simulink model "PubIfDecisionLSM_MDL"  (R2020b)
settings: configuration reference "DspaceConfig" (kept outside this file)
PostLoadFcn:
  | if any(exist('dsrtsu_mdlpostloadfcn', 'file') ~= 0), dsrtsu_mdlpostloadfcn('Execute', bdroot); end
InitFcn:
  | , if any(exist('rtifpga_mdlclblib', 'file') ~= 0), rtifpga_mdlclblib('Init', bdroot); end,
  | , if any(exist('dsmpb_private', 'file') ~= 0), dsmpb_private('dsmpb_mdlclblib', 'Init', bdroot); end,
values from neighbouring files (symbols this model uses):
  P_LSM_ALC_Enable = 0.0    [LSM_Parameter.sldd]
  P_LSM_AwayEdge_offset = 0.1    [LSM_Parameter.sldd]
  P_LSM_CentValidErr = 1.0    [LSM_Parameter.sldd]
  P_LSM_DOP_C0_EN_Limit = 0.8    [LSM_Parameter.sldd]
  P_LSM_DOP_C0_out_Limit = 2.0    [LSM_Parameter.sldd]
  P_LSM_DOP_C1_EN_Limit : value not decoded    [LSM_Parameter.sldd]
  P_LSM_DOP_C1_out_Limit : value not decoded    [LSM_Parameter.sldd]
  P_LSM_DOP_C1AndC2_Lim_X : value not decoded    [LSM_Parameter.sldd]
  P_LSM_DOP_C2_EN_Limit : value not decoded    [LSM_Parameter.sldd]
  P_LSM_DOP_C2_out_Limit : value not decoded    [LSM_Parameter.sldd]
  P_LSM_DOP_In_Pre2Dop_Dis = 1.0    [LSM_Parameter.sldd]
  P_LSM_DOP_Out_Pre2Dop_Dis = 2.0    [LSM_Parameter.sldd]
  P_LSM_DOP_PreDis_X : value not decoded    [LSM_Parameter.sldd]
  P_LSM_DOP_PreDis_Y : value not decoded    [LSM_Parameter.sldd]
  P_LSM_DOPEnableSW = 1.0    [LSM_Parameter.sldd]
  P_LSM_DOPValid_CheckTime = 0.06    [LSM_Parameter.sldd]
  P_LSM_DoubleLine_Curr2Cent_Dislimit = 0.5    [LSM_Parameter.sldd]
  P_LSM_DoubleLine_Dop2Cent_Dislimit = 0.5    [LSM_Parameter.sldd]
  P_LSM_DoubleLine_DOPOut_C1 : value not decoded    [LSM_Parameter.sldd]
  P_LSM_DoubleLine_Pre2Cent_Dislimit = 1.0    [LSM_Parameter.sldd]
  P_LSM_Error_Limit = 0.5    [LSM_Parameter.sldd]
  P_LSM_IFV2CenterAxis = 0.0    [LSM_Parameter.sldd]
  P_LSM_IFV2RearAxis = 0.0    [LSM_Parameter.sldd]
  P_LSM_Line2Edge_limit = 0.5    [LSM_Parameter.sldd]
  P_LSM_Line_Error = 0.1    [LSM_Parameter.sldd]
  P_LSM_LineSTD_Limit = 0.15    [LSM_Parameter.sldd]
  P_LSM_NOH_Switch = 0.0    [LSM_Parameter.sldd]
  P_LSM_OTL_C0_Factor = 1.0    [LSM_Parameter.sldd]
  P_LSM_OTL_C1_Factor = 0.5    [LSM_Parameter.sldd]
  P_LSM_OTL_C2_Factor = 0.5    [LSM_Parameter.sldd]
  P_LSM_Pre2OnlyLineDis = 5.0    [LSM_Parameter.sldd]
  P_LSM_Pre_t = 0.0    [LSM_Parameter.sldd]
  P_LSM_SingleLine_Cent2Edge_Dislimit = 100.0    [LSM_Parameter.sldd]
  P_LSM_SingleLine_Curr2Cent_Dislimit = 0.2    [LSM_Parameter.sldd]
  P_LSM_SingleLine_Dop2Cent_Dislimit = 0.2    [LSM_Parameter.sldd]
  P_LSM_SingleLine_DOPOut_C1 : value not decoded    [LSM_Parameter.sldd]
  P_LSM_SingleLine_Pre2Cent_Dislimit = 0.5    [LSM_Parameter.sldd]
  P_LSM_TJALimitSpd = 60.0    [LSM_Parameter.sldd]
undefined symbols (not defined in the file or in its folder): P_lCS_IFV2CenterAxis, P_LCS_IFV2RearAxis, P_LSM_EntryEdge_offset, P_LSM_EntryLnChngEnSwitch, P_LSM_EntryVanishDis, P_LSM_LinetLostTime, P_LSM_LineWijCal_C12, P_LSM_LineWijCal_C13, P_LSM_MapValid_ErrorSwitch, P_LSM_PosLineLcFac, P_LSM_SpdLim_Stub_Spd, P_LSM_SpdLim_StubLength, P_LSM_SpdTurnAlarm
libraries: simulink x324, TrueDurationTime x11
(part 10 of 25)

== system PubIfDecisionLSM_MDL/Subsystem1/TargetLineCalc_20ms2/TargetLineCalc/Subsystem3 ==
  Intersec_available : Inport  OutDataTypeStr=uint8
  f_distance : Inport  Port=2  OutDataTypeStr=single
  f_end_dis : Inport  Port=3
  en_direction : Inport  Port=4  OutDataTypeStr=uint8
  i_rec_lanes_num : Inport  Port=5  OutDataTypeStr=uint8
  i_rec_lanes : Inport  Port=6  OutDataTypeStr=uint8
  nLaneNum : Inport  Port=7  OutDataTypeStr=uint8
  nLaneID : Inport  Port=8  OutDataTypeStr=uint8
  i_mapvalid : Inport  Port=9  OutDataTypeStr=uint8
  i_on_nav_path : Inport  Port=10  OutDataTypeStr=uint8
  curr_b_vanish_valid : Inport  Port=11  OutDataTypeStr=boolean
  Exit_dDisStart : Inport  Port=12  OutDataTypeStr=single
  ExitLineExist : Inport  Port=13  OutDataTypeStr=uint8
  Exit_dC0V : Inport  Port=14  OutDataTypeStr=single
  RoadType : Inport  Port=15  OutDataTypeStr=uint8
  VehInLeftmostLane : Inport  Port=16  OutDataTypeStr=boolean
  VehInRightmostLane : Inport  Port=17  OutDataTypeStr=boolean
  Entry_bIsLineExist : Inport  Port=18
  Entry_dDisStart : Inport  Port=19
  Entry_dC0V : Inport  Port=20
  "curr_f_vanish_pt_dis " : Inport  Port=21
  currentLane_type : Inport  Port=22
  currentLane_valid : Inport  Port=23
  ChgSpd_Dis : Inport  Port=24
  SpdChgMax : Inport  Port=25
  rightLane_valid : Inport  Port=26
  rightLane_type : Inport  Port=27
  right_b_vanish_valid : Inport  Port=28
  right_f_vanish_pt_dis : Inport  Port=29
  leftLane_valid : Inport  Port=30
  leftLane_type : Inport  Port=31
  left_b_vanish_valid : Inport  Port=32
  " left_f_vanish_pt_dis" : Inport  Port=33
  RFM_ODD : Inport  Port=34  OutDataTypeStr=Bus: RFM_ODD_BUS  PortDimensions=1  BusOutputAsStruct=on
  NOH_Sts : Inport  Port=35
  vehSpd : Inport  Port=36
  Double_Line_Lost : Inport  Port=37
  HWASts : Inport  Port=38
  KapTraj : Inport  Port=39
  VxvRef : Inport  Port=40
  TarLineValid : Inport  Port=41
  TarLineA3 : Inport  Port=42
  TarLineA2 : Inport  Port=43
  TarLineA1 : Inport  Port=44
  TarLineA0 : Inport  Port=45
  Chart1 : Stateflow chart  TreatAsAtomicUnit=on
  EgoLineRef : Subsystem
  HWASts1 : InportShadow  Port=38
  Signal Copy{,1..8,13,16..17} (12 alike) : SignalConversion  OverrideOpt=off
  Subsystem : Subsystem
  Subsystem1 : Subsystem
  Subsystem2 : Subsystem
  Subsystem3 : Subsystem
  Subsystem4 : Subsystem
  Terminator : Terminator
  Unit Delay : UnitDelay  SampleTime=-1  HasFrameUpgradeWarning=on
  VehInRightmostLane1 : InportShadow  Port=17  OutDataTypeStr=boolean
  nLaneNum1 : InportShadow  Port=7  OutDataTypeStr=uint8
  nLaneNum2 : InportShadow  Port=7  OutDataTypeStr=uint8
  PilotRoadSts : Outport  OutDataTypeStr=uint8
  PilotTurnSwSts : Outport  Port=2  OutDataTypeStr=uint8
  PilotSts : Outport  Port=3  OutDataTypeStr=uint8
  LaneChange : Outport  Port=4  OutDataTypeStr=uint8
  LSM_PilotSPL : Outport  Port=5  OutDataTypeStr=uint8
  PilotSPLDist : Outport  Port=6  OutDataTypeStr=uint16
  LSM_PilotNohExitDist : Outport  Port=7
  NOH_HMI_Voice : Outport  Port=8
  wires:
  SpdChgMax/1 -> Subsystem/45(SpdChgMax)
  ChgSpd_Dis/1 -> Subsystem/44(ChgSpd_Dis)
  Signal Copy8/1 -> Subsystem2/7(VehInRightmostLane)
  Signal Copy7/1 -> Chart1/6(vehSpd)  "LSM_VehSpd_HiFlag"
  Signal Copy6/1 -> Subsystem4/11(LaneNum)
  Chart1/3(m) -> Terminator/1  "LSM_TurnHighSpdFlag"
  HWASts1/1 -> Subsystem2/31(HWASts)
  EgoLineRef/1(LaneChangeEnable) -> Subsystem/48(LaneChangeEnable)
  TarLineA0/1 -> EgoLineRef/7(TarLineA0)
  TarLineA1/1 -> EgoLineRef/6(TarLineA1)
  TarLineA2/1 -> EgoLineRef/5(TarLineA2)
  TarLineA3/1 -> EgoLineRef/4(TarLineA3)
  TarLineValid/1 -> EgoLineRef/3(TarLineValid)
  VxvRef/1 -> EgoLineRef/2(VxvRef)
  KapTraj/1 -> EgoLineRef/1(KapTraj)
  Subsystem2/36(EntryStubVanishTurn) -> Subsystem/41(EntryStubVanishTurn)
  [f_distance] -> Subsystem/4(f_distance)
  [f_distance] -> Subsystem1/5(f_distance)
  Subsystem4/1(NOH_HMI_Voice) -> NOH_HMI_Voice/1
  HWASts/1 -> Subsystem4/14(HWASts)
  [NoPUCR_Dis] -> Subsystem4/13(NoPUCR_Dis)
  [NoPUCR] -> Subsystem4/12(NoPUCR)
  nLaneNum1/1 -> Signal Copy6/1
  Double_Line_Lost/1 -> Subsystem4/10(Double_Line_Lost)
  [f_distance] -> Subsystem4/9(f_distance)
  [rExitStub4_takeover] -> Subsystem4/8(rExitStub4_takeover)
  [lExitStub4_takeover] -> Subsystem4/7(lExitStub4_takeover)
  [exitTakeOverValid] -> Subsystem4/6(exitTakeOverValid)
  [b_vanish_valid] -> Subsystem4/5(b_vanish_valid)
  [changeVoice] -> Subsystem4/4(changeVoice)
  [f_vanish_pt_dis] -> Subsystem4/3(f_vanish_pt_dis)
  [en_direction] -> Subsystem4/2(en_direction)
  [PilotRoadSts] -> Subsystem4/1(PilotRoadSts)
  [NoPUCR] -> Subsystem1/4(NoPUCR)
  Subsystem2/35(StudLengthSpd) -> Subsystem/40(StudLengthSpd)
  [vehSpd] -> Subsystem/47(vehSpd)
  Subsystem2/34(ForbidActive) -> Subsystem/39(ForbidActive)
  currentLane_valid/1 -> Subsystem2/30(currentLane_valid)
  Subsystem2/33(DecSpd) -> Subsystem/38(DecSpd)
  Subsystem/8(NoPUCR_Dis) -> [NoPUCR_Dis]
  Subsystem/7(NoPUCR) -> [NoPUCR]
  Subsystem2/37(exitTakeOverValid) -> [exitTakeOverValid]
  [vehSpd] -> Signal Copy7/1
  Signal Copy13/1 -> Subsystem/42(RFM_ODD)
  Signal Copy17/1 -> Subsystem2/23(VehSpd), [vehSpd]
  Signal Copy16/1 -> Chart1/5(nLaneNum)  "LSM_nLaneNum_HiFlag"
  Signal Copy5/1 -> Chart1/4(VehInRightmostLane)  "LSM_MostLaneRight_HiFlag"
  Subsystem/1(PilotRoadSts) -> PilotRoadSts/1, Chart1/1(PilotRoadSts), Unit Delay/1, [PilotRoadSts]
  Chart1/2(changeVoice) -> [changeVoice]
  vehSpd/1 -> Signal Copy17/1
  nLaneNum2/1 -> Signal Copy16/1
  VehInRightmostLane1/1 -> Signal Copy5/1
  Unit Delay/1 -> Chart1/2(PilotRoadSts_K)
  Chart1/1(PilotTurnSwSts) -> PilotTurnSwSts/1, [PilotTurnSwSts]
  Subsystem2/32(roadClass) -> Subsystem/37(roadClass)
  currentLane_type/1 -> Subsystem2/22(currentLane_type)
  leftLane_type/1 -> Subsystem2/21(leftLane_type)
  rightLane_type/1 -> Subsystem2/19(rightLane_type)
  Subsystem/6(LSM_PilotNohExitDist) -> LSM_PilotNohExitDist/1
  RFM_ODD/1 -> Signal Copy13/1
  leftLane_valid/1 -> Subsystem2/20(leftLane_valid)
  rightLane_valid/1 -> Subsystem2/18(rightLane_valid)
  Subsystem2/31(turndir) -> Subsystem/36(turndir)
  Signal Copy2/1 -> Subsystem2/1(Exit_bIsLineExist), Subsystem/5(bIsLineExist)
  Signal Copy4/1 -> [f_distance], Subsystem2/2(f_distance)
  Signal Copy3/1 -> Subsystem1/3(RoadType)
  Signal Copy1/1 -> Subsystem1/2(i_on_nav_path)
  Signal Copy/1 -> Subsystem1/1(i_mapvalid)
  f_distance/1 -> Signal Copy4/1
  RoadType/1 -> Signal Copy3/1
  [nLaneID] -> Subsystem3/2(nLaneID)
  [PilotTurnSwSts] -> Subsystem3/1(PilotTurnSwSts)
  Subsystem/5(PilotSts) -> PilotSts/1
  Subsystem2/30(Vanish_turnleft_takeover) -> Subsystem/35(Vanish_turnleft_takeover)
  Subsystem2/29(EntryStub5_takeover) -> Subsystem/34(EntryStub5_takeover)  "LSM_EntryStub5_takeover"
  Subsystem2/28(lExitStub4_takeover) -> [lExitStub4_takeover], Subsystem/33(lExitStub4_takeover)
  Subsystem2/27(rExitStub4_takeover) -> Subsystem/32(rExitStub4_takeover), [rExitStub4_takeover]
  Subsystem3/1(LaneChange) -> LaneChange/1
  "curr_f_vanish_pt_dis "/1 -> Subsystem2/17(" curr_f_vanish_pt_dis "), [f_vanish_pt_dis]
  Subsystem/4(PilotSPLDist) -> PilotSPLDist/1
  Subsystem/3(LSM_PilotSPL) -> LSM_PilotSPL/1
  Subsystem2/26(EntryStub5_TurnLeft) -> Subsystem/31(EntryStub5_TurnLeft)
  Subsystem2/25(EntryStub6) -> Subsystem/30(EntryStub6)  "LSM_EntryStub6"
  Subsystem2/24(EntryStub5) -> Subsystem/29(EntryStub5)  "LSM_EntryStub5"
  Subsystem2/23(EntryStub4) -> Subsystem/28(EntryStub4)  "LSM_EntryStub4"
  Subsystem2/22(EntryStub3) -> Subsystem/27(EntryStub3)  "LSM_EntryStub3"
  Subsystem2/21(EntryStub2) -> Subsystem/26(EntryStub2)  "LSM_EntryStub2"
  Subsystem2/20(OneLane) -> Subsystem/25(OneLane)  "LSM_OneLane"
  Subsystem2/19(Forbid_TurnLeft) -> Subsystem/24(FrbLeft)
  Subsystem2/18(Forbid_TurnRight) -> Subsystem/23(FrbRight)
  Subsystem2/17(CruiseTurn) -> Subsystem/22(CruiseTurn)  "LSM_CruiseTurn"
  Subsystem2/15(lExitStub2) -> Subsystem/20(lExitStub2)  "LSM_IExitStub2"
  Subsystem2/14(lExitStub1) -> Subsystem/19(lExitStub1)  "LSM_IExitStub1"
  Subsystem2/13(CruiseLeft) -> Subsystem/18(CruiseLeft)  "LSM_CruiseLeft"
  Subsystem2/12(CruiseRight) -> Subsystem/17(CruiseRight)  "LSM_CruiseRight"
  Subsystem2/11(EntryStub1) -> Subsystem/16(EntryStub1)  "LSM_EntryStub1"
  Subsystem2/10(Vanish_turnleft) -> Subsystem/15(Vanish_turnleft)  "LSM_Vanish_turnleft"
  Subsystem2/8(rExitStub2) -> Subsystem/13(rExitStub2)  "LSM_rExitStub2"
  Subsystem2/7(rExitStub1) -> Subsystem/12(rExitStub1)  "LSM_rExitStub1"
  Subsystem2/6(TurnRight) -> Subsystem/11(TurnRight)  "LSM_TurnRight"
  Subsystem2/5(TurnLeft) -> Subsystem/10(TurnLeft)  "LSM_TurnLeft"
  Subsystem2/4(CruiseValid) -> Subsystem/9(CruiseValid)  "LSM_CruiseValid"
  Subsystem2/3(LeftStub) -> Subsystem/8(LeftStub)  "LSM_LeftStub"
  Subsystem2/2(RightStub) -> Subsystem/7(RightStub)  "LSM_RightStub"
  Subsystem2/1(StubValid) -> Subsystem/6(StubValid)  "LSM_StubValid"
  Subsystem/2(PilotTurnSwSts) -> Chart1/3(PilotTurnSwSts_Init)
  Entry_dC0V/1 -> [Entry_dC0V], Subsystem2/16(Entry_dC0V)
  Entry_dDisStart/1 -> Subsystem2/15(Entry_dDisStart)
  Entry_bIsLineExist/1 -> Subsystem2/14(Entry_bIsLineExist)
  Intersec_available/1 -> Subsystem2/3(b_is_available)
  Subsystem2/16(lExitStub3) -> Subsystem/21(lExitStub3)  "LSM_IExitStub3"
  en_direction/1 -> Subsystem2/6(en_direction), [en_direction]
  ExitLineExist/1 -> Signal Copy2/1
  i_rec_lanes/1 -> Subsystem2/4(i_rec_lanes)
  i_mapvalid/1 -> Signal Copy/1
  i_rec_lanes_num/1 -> Subsystem2/10(i_rec_lanes_num)
  Subsystem2/9(rExitStub3) -> Subsystem/14(rExitStub3)  "LSM_rExitStub3"
  Exit_dDisStart/1 -> Subsystem2/12(" Exit_dDisStart")
  Exit_dC0V/1 -> Subsystem2/13(Exit_dC0V)
  i_on_nav_path/1 -> Signal Copy1/1
  nLaneID/1 -> Subsystem2/5(nLaneID), [nLaneID]
  VehInRightmostLane/1 -> Signal Copy8/1
  VehInLeftmostLane/1 -> Subsystem2/8(VehInLeftmostLane)
  nLaneNum/1 -> Subsystem2/9(nLaneNum)
  curr_b_vanish_valid/1 -> Subsystem2/11(" curr_b_vanish_valid"), [b_vanish_valid]
  f_end_dis/1 -> Subsystem2/24(f_end_dis)
  [PilotRoadSts] -> Subsystem2/25(PilotRoadSts)
  left_b_vanish_valid/1 -> Subsystem2/26(left_b_vanish_valid)
  " left_f_vanish_pt_dis"/1 -> Subsystem2/27(" left_f_vanish_pt_dis")
  right_b_vanish_valid/1 -> Subsystem2/28(right_b_vanish_valid)
  right_f_vanish_pt_dis/1 -> Subsystem2/29(right_f_vanish_pt_dis)
  Subsystem1/1(i_mapvalid_out) -> Subsystem/1(i_mapvalid)
  Subsystem1/2(i_on_nav_path_out) -> Subsystem/2(i_on_nav_path)
  Subsystem1/3(RoadType_out) -> Subsystem/3(RoadType)
  NOH_Sts/1 -> Subsystem/43(NOH_Sts)
  [Entry_dC0V] -> Subsystem/46(Entry_dC0V)

== system PubIfDecisionLSM_MDL/Subsystem1/TargetLineCalc_20ms2/TargetLineCalc/TypeConf ==
  LeftType : Inport
  LeftDLMType : Inport  Port=2
  LeftDECELType : Inport  Port=3
  RightType : Inport  Port=4
  RightDLMType : Inport  Port=5
  RightDECELType : Inport  Port=6
  RoadWidthCalc1 : MATLAB Function  TreatAsAtomicUnit=on
  Unit Delay36 : UnitDelay  SampleTime=-1  HasFrameUpgradeWarning=on
  Unit Delay37 : UnitDelay  SampleTime=-1  HasFrameUpgradeWarning=on
  Out1 : Outport
  Out2 : Outport  Port=2
  wires:
  RightDECELType/1 -> RoadWidthCalc1/6(RightDECELType)
  LeftDECELType/1 -> RoadWidthCalc1/3(LeftDECELType)
  RightDLMType/1 -> RoadWidthCalc1/5(RightDLMType)
  LeftDLMType/1 -> RoadWidthCalc1/2(LeftDLMType)
  RightType/1 -> RoadWidthCalc1/4(RightType)
  Unit Delay36/1 -> RoadWidthCalc1/8(Cnt2K1)
  RoadWidthCalc1/2(RightEn) -> Out2/1
  LeftType/1 -> RoadWidthCalc1/1(LeftType)
  RoadWidthCalc1/4(Cnt2) -> Unit Delay36/1
  RoadWidthCalc1/3(Cnt1) -> Unit Delay37/1
  Unit Delay37/1 -> RoadWidthCalc1/7(Cnt1K1)
  RoadWidthCalc1/1(LeftEn) -> Out1/1

== system PubIfDecisionLSM_MDL/Subsystem1/TargetLineCalc_20ms2/TargetLineCalc/TypeConf1 ==
  LeftType : Inport
  RightType : Inport  Port=2
  RoadWidthCalc1 : MATLAB Function  TreatAsAtomicUnit=on
  Unit Delay36 : UnitDelay  SampleTime=-1  HasFrameUpgradeWarning=on
  Unit Delay37 : UnitDelay  SampleTime=-1  HasFrameUpgradeWarning=on
  LeftEn : Outport
  RightEn : Outport  Port=2
  wires:
  RoadWidthCalc1/1(LeftEn) -> LeftEn/1
  Unit Delay37/1 -> RoadWidthCalc1/3(Cnt1K1)
  RoadWidthCalc1/3(Cnt1) -> Unit Delay37/1
  RoadWidthCalc1/4(Cnt2) -> Unit Delay36/1
  LeftType/1 -> RoadWidthCalc1/1(LeftType)
  RoadWidthCalc1/2(RightEn) -> RightEn/1
  Unit Delay36/1 -> RoadWidthCalc1/4(Cnt2K1)
  RightType/1 -> RoadWidthCalc1/2(RightType)

== system PubIfDecisionLSM_MDL/Subsystem1/TargetLineCalc_20ms/TargetLineCalc/Subsystem3/Subsystem ==
  note: b_is_available
  i_mapvalid : Inport
  i_on_nav_path : Inport  Port=2
  RoadType : Inport  Port=3
  bIsLineExist : Inport  Port=4
  f_distance : Inport  Port=5
  StubValid : Inport  Port=6
  RightStub : Inport  Port=7
  LeftStub : Inport  Port=8
  CruiseValid : Inport  Port=9
  TurnLeft : Inport  Port=10
  TurnRight : Inport  Port=11
  rExitStub1 : Inport  Port=12
  rExitStub2 : Inport  Port=13
  rExitStub3 : Inport  Port=14
  Vanish_turnleft : Inport  Port=15
  EntryStub1 : Inport  Port=16
  CruiseRight : Inport  Port=17
  CruiseLeft : Inport  Port=18
  lExitStub1 : Inport  Port=19
  lExitStub2 : Inport  Port=20
  lExitStub3 : Inport  Port=21
  CruiseTurn : Inport  Port=22
  FrbRight : Inport  Port=23
  FrbLeft : Inport  Port=24
  OneLane : Inport  Port=25
  EntryStub2 : Inport  Port=26
  EntryStub3 : Inport  Port=27
  EntryStub4 : Inport  Port=28
  EntryStub5 : Inport  Port=29
  EntryStub6 : Inport  Port=30
  EntryStub5_TurnLeft : Inport  Port=31
  rExitStub4_takeover : Inport  Port=32
  lExitStub4_takeover : Inport  Port=33
  EntryStub5_takeover : Inport  Port=34
  Vanish_turnleft_takeover : Inport  Port=35
  Chart : Stateflow chart  TreatAsAtomicUnit=on
  Chart1 : Stateflow chart  TreatAsAtomicUnit=on
  Compare To Constant1 : simulink/Logic and Bit Operations/Compare To Constant  relop=>  const=0  OutDataTypeStr=boolean
  Compare To Constant12 : simulink/Logic and Bit Operations/Compare To Constant  relop===  const=3  OutDataTypeStr=boolean
  Constant3 : Constant  Value=100  OutDataTypeStr=uint16
  Logical Operator6 : Logic  AllPortsSameDT=off  OutDataTypeStr=boolean
  MATLAB Function : MATLAB Function  TreatAsAtomicUnit=on
  Subtract : Sum  Inputs=+-
  PilotRoadSts : Outport
  PilotTurnSwSts : Outport  Port=2
  LSM_PilotSPL : Outport  Port=3
  PilotSPLDist : Outport  Port=4
  PilotSts : Outport  Port=5
  wires:
  Chart1/2(PilotTurnSwSts) -> PilotTurnSwSts/1
  f_distance/1 -> Subtract/1
  [rExitStub3] -> Chart/4(rExitStub3)
  lExitStub3/1 -> [lExitStub3], Chart1/21(lExitStub3)
  Subtract/1 -> Chart1/16(f_distance)
  EntryStub5/1 -> Chart1/28(EntryStub5)
  FrbRight/1 -> Chart1/24(FrbRight)
  Chart1/1(PilotRoadSts) -> Chart/1(PilotRoadSts_init)
  [lExitStub3] -> Chart/3(lExitStub3)
  TurnLeft/1 -> Chart1/6(TurnLeft)
  Constant3/1 -> Subtract/2
  rExitStub2/1 -> Chart1/11(rExitStub2)
  EntryStub1/1 -> Chart1/9(EntryStub1)
  Chart/1(PilotRoadSts) -> PilotRoadSts/1
  rExitStub1/1 -> Chart1/10(rExitStub1)
  CruiseValid/1 -> Chart1/5(CruiseValid)
  bIsLineExist/1 -> Chart/2(bIsLineExist)
  EntryStub6/1 -> Chart1/29(EntryStub6)
  lExitStub1/1 -> Chart1/19(lExitStub1)
  RightStub/1 -> Chart1/2(RightStub)
  LeftStub/1 -> Chart1/4(LeftStub)
  Vanish_turnleft/1 -> Chart1/8(Vanish_turnleft)
  CruiseRight/1 -> Chart1/15(CruiseRight)
  FrbLeft/1 -> Chart1/23(FrbLeft)
  OneLane/1 -> Chart1/25(OneLane)
  EntryStub3/1 -> Chart1/26(EntryStub3)
  EntryStub4/1 -> Chart1/27(EntryStub4)
  CruiseLeft/1 -> Chart1/14(CruiseLeft)
  EntryStub5_TurnLeft/1 -> Chart1/30(EntryStub5_TurnLeft)
  StubValid/1 -> Chart1/1(StubValid)
  Chart1/3(LSM_PilotSPL) -> LSM_PilotSPL/1
  CruiseTurn/1 -> Chart1/17(CruiseTurn)
  Chart1/4(PilotSPLDist) -> PilotSPLDist/1
  rExitStub3/1 -> [rExitStub3], Chart1/22(rExitStub3)
  TurnRight/1 -> Chart1/7(TurnRight)
  lExitStub2/1 -> Chart1/20(lExitStub2)
  i_on_nav_path/1 -> Chart1/13(i_on_nav_path)
  EntryStub2/1 -> Chart1/18(EntryStub2)
  Compare To Constant12/1 -> Logical Operator6/1
  Compare To Constant1/1 -> Logical Operator6/2
  MATLAB Function/1(PilotSts) -> PilotSts/1
  RoadType/1 -> MATLAB Function/2(RoadType), Compare To Constant1/1, Chart1/3(RoadType)
  Logical Operator6/1 -> MATLAB Function/1(NOH_Valid)
  i_mapvalid/1 -> Chart1/12(i_mapvalid), Compare To Constant12/1
  rExitStub4_takeover/1 -> MATLAB Function/3(rExitStub4_takeover)
  lExitStub4_takeover/1 -> MATLAB Function/4(lExitStub4_takeover)
  EntryStub5_takeover/1 -> MATLAB Function/5(EntryStub5_takeover)
  Vanish_turnleft_takeover/1 -> MATLAB Function/6(Vanish_turnleft_takeover)
